simulink model "SWC_HALOUT_type"  (R2021b)
settings: Solver=FixedStepDiscrete  StartTime=0.0  StopTime=10.0  FixedStep=0.005  RelTol=1e-3
undefined symbols (not defined in the file): DIDLen_APPD, DIDLen_APPE, DIDLen_APPPedalZP, DIDLen_APSFunConfig, DIDLen_AutoLock, DIDLen_AutoWipHSpdEN, DIDLen_CALID, DIDLen_CDEODT, DIDLen_CLRDIST, DIDLen_DKCBLESta, DIDLen_DKCKey, DIDLen_DKCSta, DIDLen_DoorNFCAnchorSta, DIDLen_DRLDis, DIDLen_DynoMode, DIDLen_ECUNAME, DIDLen_FDDKCCoordXY, DIDLen_FMHTimer, DIDLen_LFLowPresThre, DIDLen_LFSensorID, DIDLen_LIDAAnchorSta, DIDLen_LRLowPresThre, DIDLen_LRSensorID, DIDLen_MILDIST, DIDLen_NUMPSATRIPSFLTMEMCLR, DIDLen_NVMPedalZP, DIDLen_OBDReq, DIDLen_ODOMETER, DIDLen_PKE, DIDLen_ProtocolId, DIDLen_PSA, DIDLen_QTYPSATRIPS, DIDLen_RFLowPresThre, DIDLen_RFSensorID, DIDLen_RRLowPresThre, DIDLen_RRSensorID, DIDLen_RUNTM, DIDLen_SensorMode, DIDLen_TestGroup, DIDLen_TireSize, DIDLen_TPMSLearnSta, DIDLen_TurnLampFLThreCurr, DIDLen_TurnLampFRThreCurr, DIDLen_TurnLampRLThreCurr, DIDLen_TurnLampRRThreCurr, DIDLen_UIDSta, DIDLen_USSConfig, DIDLen_UWBAnchorSta, DIDLen_VIN, DIDLen_VSS, DIDLen_WhlPres, DIDLen_WhlSensorBattSta, DIDLen_WhlTmp, DIDLen_WipRLSCmdCutFilter, DIDLen_WipRLSCmdHoldFilter, DIDLen_XWDMode, DIDNum_APPD, DIDNum_APPE, DIDNum_APPPedalZP, DIDNum_APSFunConfig ... (+504)
libraries: simulink x893, FVT_lib x320, hdlsllib x6, hcu_lib x5, halout x1
(part 2 of 11)

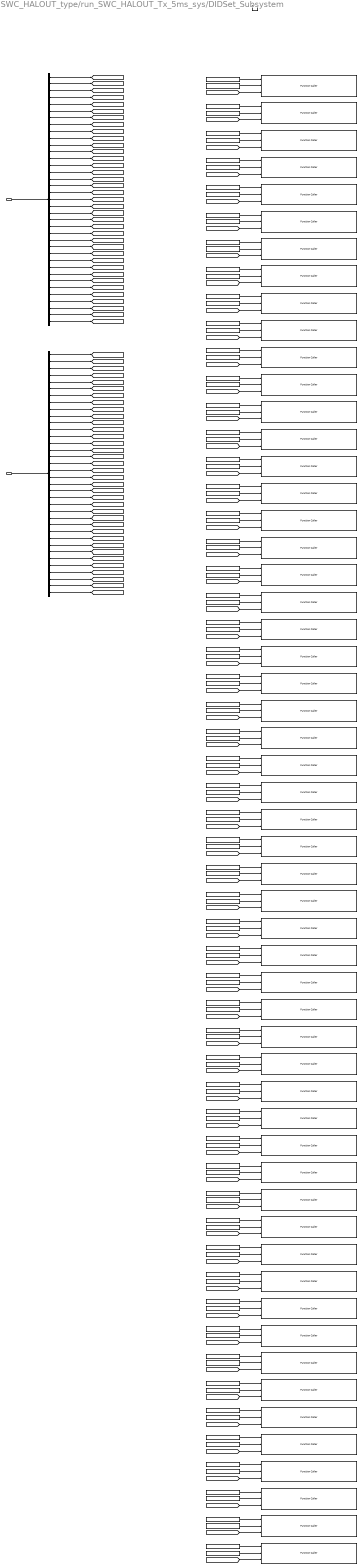
== system SWC_HALOUT_type/run_SWC_HALOUT_Tx_5ms_sys/DIDSet_Subsystem ==
  BOUTP_DIDSetData_outputs : Inport
  BHAL_DID_outputs : Inport  Port=2
  trig_SetDID : TriggerPort  TriggerType=function-call  VariantControl=(inherit)  PortDimensions=1
  DIDLen : Constant  Value=DIDNum_XWDMode
  DIDLen1 : Constant  Value=DIDNum_DKCKey
  DIDLen10 : Constant  Value=DIDNum_DRLDis
  DIDLen11 : Constant  Value=DIDNum_AutoWipHSpdEN
  DIDLen12 : Constant  Value=DIDNum_WipRLSCmdHoldFilter
  DIDLen13 : Constant  Value=DIDNum_WipRLSCmdCutFilter
  DIDLen14 : Constant  Value=DIDNum_LFSensorID
  DIDLen15 : Constant  Value=DIDNum_RFSensorID
  DIDLen16 : Constant  Value=DIDNum_LRSensorID
  DIDLen17 : Constant  Value=DIDNum_RRSensorID
  DIDLen18 : Constant  Value=DIDNum_WhlPres
  DIDLen19 : Constant  Value=DIDNum_WhlTmp
  DIDLen2 : Constant  Value=DIDNum_DynoMode
  DIDLen20 : Constant  Value=DIDNum_WhlSensorBattSta
  DIDLen21 : Constant  Value=DIDNum_LFLowPresThre
  DIDLen22 : Constant  Value=DIDNum_RFLowPresThre
  DIDLen23 : Constant  Value=DIDNum_LRLowPresThre
  DIDLen24 : Constant  Value=DIDNum_RRLowPresThre
  DIDLen25 : Constant  Value=DIDNum_SensorMode
  DIDLen26 : Constant  Value=DIDNum_TPMSLearnSta
  DIDLen27 : Constant  Value=DIDNum_USSConfig
  DIDLen28 : Constant  Value=DIDNum_TireSize
  DIDLen29 : Constant  Value=DIDNum_APSFunConfig
  DIDLen3 : Constant  Value=DIDNum_APPPedalZP
  DIDLen30 : Constant  Value=DIDNum_VSS
  DIDLen31 : Constant  Value=DIDNum_OBDReq
  DIDLen32 : Constant  Value=DIDNum_RUNTM
  DIDLen33 : Constant  Value=DIDNum_MILDIST
  DIDLen34 : Constant  Value=DIDNum_CLRDIST
  DIDLen35 : Constant  Value=DIDNum_APPD
  DIDLen36 : Constant  Value=DIDNum_APPE
  DIDLen37 : Constant  Value=DIDNum_ODOMETER
  DIDLen38 : Constant  Value=DIDNum_NUMPSATRIPSFLTMEMCLR
  DIDLen39 : Constant  Value=DIDNum_VIN
  DIDLen4 : Constant  Value=DIDNum_TurnLampFRThreCurr
  DIDLen40 : Constant  Value=DIDNum_CALID
  DIDLen41 : Constant  Value=DIDNum_ECUNAME
  DIDLen42 : Constant  Value=DIDNum_ProtocolId
  DIDLen43 : Constant  Value=DIDNum_TestGroup
  DIDLen44 : Constant  Value=DIDNum_PSA
  DIDLen45 : Constant  Value=DIDNum_PKE
  DIDLen46 : Constant  Value=DIDNum_CDEODT
  DIDLen47 : Constant  Value=DIDNum_QTYPSATRIPS
  DIDLen48 : Constant  Value=DIDNum_DKCSta
  DIDLen49 : Constant  Value=DIDNum_DKCBLESta
  DIDLen5 : Constant  Value=DIDNum_TurnLampRRThreCurr
  DIDLen50 : Constant  Value=DIDNum_UWBAnchorSta
  DIDLen51 : Constant  Value=DIDNum_LIDAAnchorSta
  DIDLen52 : Constant  Value=DIDNum_DoorNFCAnchorSta
  DIDLen53 : Constant  Value=DIDNum_UIDSta
  DIDLen54 : Constant  Value=DIDNum_FDDKCCoordXY
  DIDLen6 : Constant  Value=DIDNum_TurnLampFLThreCurr
  DIDLen7 : Constant  Value=DIDNum_TurnLampRLThreCurr
  DIDLen8 : Constant  Value=DIDNum_FMHTimer
  DIDLen9 : Constant  Value=DIDNum_AutoLock
  DIDNum : Constant  Value=DIDLen_XWDMode
  DIDNum1 : Constant  Value=DIDLen_DKCKey
  DIDNum10 : Constant  Value=DIDLen_DRLDis
  DIDNum11 : Constant  Value=DIDLen_AutoWipHSpdEN
  DIDNum12 : Constant  Value=DIDLen_WipRLSCmdHoldFilter
  DIDNum13 : Constant  Value=DIDLen_WipRLSCmdCutFilter
  DIDNum14 : Constant  Value=DIDLen_LFSensorID
  DIDNum15 : Constant  Value=DIDLen_RFSensorID
  DIDNum16 : Constant  Value=DIDLen_LRSensorID
  DIDNum17 : Constant  Value=DIDLen_RRSensorID
  DIDNum18 : Constant  Value=DIDLen_WhlPres
  DIDNum19 : Constant  Value=DIDLen_WhlTmp
  DIDNum2 : Constant  Value=DIDLen_DynoMode
  DIDNum20 : Constant  Value=DIDLen_WhlSensorBattSta
  DIDNum21 : Constant  Value=DIDLen_LFLowPresThre
  DIDNum22 : Constant  Value=DIDLen_RFLowPresThre
  DIDNum23 : Constant  Value=DIDLen_LRLowPresThre
  DIDNum24 : Constant  Value=DIDLen_RRLowPresThre
  DIDNum25 : Constant  Value=DIDLen_SensorMode
  DIDNum26 : Constant  Value=DIDLen_TPMSLearnSta
  DIDNum27 : Constant  Value=DIDLen_USSConfig
  DIDNum28 : Constant  Value=DIDLen_TireSize
  DIDNum29 : Constant  Value=DIDLen_APSFunConfig
  DIDNum3 : Constant  Value=DIDLen_APPPedalZP
  DIDNum30 : Constant  Value=DIDLen_VSS
  DIDNum31 : Constant  Value=DIDLen_OBDReq
  DIDNum32 : Constant  Value=DIDLen_RUNTM
  DIDNum33 : Constant  Value=DIDLen_MILDIST
  DIDNum34 : Constant  Value=DIDLen_CLRDIST
  DIDNum35 : Constant  Value=DIDLen_APPD
  DIDNum36 : Constant  Value=DIDLen_APPE
  DIDNum37 : Constant  Value=DIDLen_ODOMETER
  DIDNum38 : Constant  Value=DIDLen_NUMPSATRIPSFLTMEMCLR
  DIDNum39 : Constant  Value=DIDLen_VIN
  DIDNum4 : Constant  Value=DIDLen_TurnLampFRThreCurr
  DIDNum40 : Constant  Value=DIDLen_CALID
  DIDNum41 : Constant  Value=DIDLen_ECUNAME
  DIDNum42 : Constant  Value=DIDLen_ProtocolId
  DIDNum43 : Constant  Value=DIDLen_TestGroup
  DIDNum44 : Constant  Value=DIDLen_PSA
  DIDNum45 : Constant  Value=DIDLen_PKE
  DIDNum46 : Constant  Value=DIDLen_CDEODT
  DIDNum47 : Constant  Value=DIDLen_QTYPSATRIPS
  DIDNum48 : Constant  Value=DIDLen_DKCSta
  DIDNum49 : Constant  Value=DIDLen_DKCBLESta
  DIDNum5 : Constant  Value=DIDLen_TurnLampRRThreCurr
  DIDNum50 : Constant  Value=DIDLen_UWBAnchorSta
  DIDNum51 : Constant  Value=DIDLen_LIDAAnchorSta
  DIDNum52 : Constant  Value=DIDLen_DoorNFCAnchorSta
  DIDNum53 : Constant  Value=DIDLen_UIDSta
  DIDNum54 : Constant  Value=DIDLen_FDDKCCoordXY
  DIDNum6 : Constant  Value=DIDLen_TurnLampFLThreCurr
  DIDNum7 : Constant  Value=DIDLen_TurnLampRLThreCurr
  DIDNum8 : Constant  Value=DIDLen_FMHTimer
  DIDNum9 : Constant  Value=DIDLen_AutoLock
  R_DIDWriteCDD_CSOP_DIDSet_APPD : FunctionCaller  FunctionPrototype=R_DIDWriteCDD_CSOP_DIDSet_APPD(u16_DIDNum_APPD,u16_DIDLen_APPD,u8_APPD)  InputArgumentSpecifications=uint16(1), uint16(1), uint8(1)
  R_DIDWriteCDD_CSOP_DIDSet_APPE : FunctionCaller  FunctionPrototype=R_DIDWriteCDD_CSOP_DIDSet_APPE(u16_DIDNum_APPE,u16_DIDLen_APPE,u8_APPE)  InputArgumentSpecifications=uint16(1), uint16(1), uint8(1)
  R_DIDWriteCDD_CSOP_DIDSet_APPPedalZP : FunctionCaller  FunctionPrototype=R_DIDWriteCDD_CSOP_DIDSet_APPPedalZP(u16_DIDNum_APPPedalZP,u16_DIDLen_APPPedalZP,u8Array3_APPPedalZP)  InputArgumentSpecifications=uint16(1), uint16(1), uint8([1;1;1])
  R_DIDWriteCDD_CSOP_DIDSet_APSFunConfig : FunctionCaller  FunctionPrototype=R_DIDWriteCDD_CSOP_DIDSet_APSFunConfig(u16_DIDNum_APSFunConfig,u16_DIDLen_APSFunConfig,u8Array16_APSFunConfig)  InputArgumentSpecifications=uint16(1), uint16(1), uint8([1;1;1;1;1;1;1;1;1;1;1;1;1;1;1;1])
  R_DIDWriteCDD_CSOP_DIDSet_AutoLock : FunctionCaller  FunctionPrototype=R_DIDWriteCDD_CSOP_DIDSet_AutoLock(u16_DIDNum_AutoLock,u16_DIDLen_AutoLock,u8_AutoLock)  InputArgumentSpecifications=uint16(1), uint16(1), uint8(1)
  R_DIDWriteCDD_CSOP_DIDSet_AutoWipHSpdEN : FunctionCaller  FunctionPrototype=R_DIDWriteCDD_CSOP_DIDSet_AutoWipHSpdEN(u16_DIDNum_AutoWipHSpdEN,u16_DIDLen_AutoWipHSpdEN,u8_AutoWipHSpdEN)  InputArgumentSpecifications=uint16(1), uint16(1), uint8(1)
  R_DIDWriteCDD_CSOP_DIDSet_CALID : FunctionCaller  FunctionPrototype=R_DIDWriteCDD_CSOP_DIDSet_CALID(u16_DIDNum_CALID,u16_DIDLen_CALID,u8Array16_CALID)  InputArgumentSpecifications=uint16(1), uint16(1), uint8([1;1;1;1;1;1;1;1;1;1;1;1;1;1;1;1])
  R_DIDWriteCDD_CSOP_DIDSet_CDEODT : FunctionCaller  FunctionPrototype=R_DIDWriteCDD_CSOP_DIDSet_CDEODT(u16_DIDNum_CDEODT,u16_DIDLen_CDEODT,u8Array8_CDEODT)  InputArgumentSpecifications=uint16(1), uint16(1), uint8([1;1;1;1;1;1;1;1])
  R_DIDWriteCDD_CSOP_DIDSet_CLRDIST : FunctionCaller  FunctionPrototype=R_DIDWriteCDD_CSOP_DIDSet_CLRDIST(u16_DIDNum_CLRDIST,u16_DIDLen_CLRDIST,u8Array2_CLRDIST)  InputArgumentSpecifications=uint16(1), uint16(1), uint8([1;1])
  R_DIDWriteCDD_CSOP_DIDSet_DKCBLESta : FunctionCaller  FunctionPrototype=R_DIDWriteCDD_CSOP_DIDSet_DKCBLESta(u16_DIDNum_DKCBLESta,u16_DIDLen_DKCBLESta,u8Array2_DKCBLESta)  InputArgumentSpecifications=uint16(1), uint16(1), uint8([1;1])
  R_DIDWriteCDD_CSOP_DIDSet_DKCKey : FunctionCaller  FunctionPrototype=R_DIDWriteCDD_CSOP_DIDSet_DKCKey(u16_DIDNum_DKCKey,u16_DIDLen_DKCKey,u8Array8_DKCKey)  InputArgumentSpecifications=uint16(1), uint16(1), uint8([1;1;1;1;1;1;1;1])
  R_DIDWriteCDD_CSOP_DIDSet_DKCSta : FunctionCaller  FunctionPrototype=R_DIDWriteCDD_CSOP_DIDSet_DKCSta(u16_DIDNum_DKCSta,u16_DIDLen_DKCSta,u8Array2_DKCSta)  InputArgumentSpecifications=uint16(1), uint16(1), uint8([1;1])
  R_DIDWriteCDD_CSOP_DIDSet_DRLDis : FunctionCaller  FunctionPrototype=R_DIDWriteCDD_CSOP_DIDSet_DRLDis(u16_DIDNum_DRLDis,u16_DIDLen_DRLDis,u8_DRLDis)  InputArgumentSpecifications=uint16(1), uint16(1), uint8(1)
  R_DIDWriteCDD_CSOP_DIDSet_DoorNFCAnchorSta : FunctionCaller  FunctionPrototype=R_DIDWriteCDD_CSOP_DIDSet_DoorNFCAnchorSta(u16_DIDNum_DoorNFCAnchorSta,u16_DIDLen_DoorNFCAnchorSta,u8Array21_DoorNFCAnchorSta)  InputArgumentSpecifications=uint16(1), uint16(1), uint8([1;1;1;1;1;1;1;1;1;1;1;1;1;1;1;1;1;1;1;1;1])
  R_DIDWriteCDD_CSOP_DIDSet_DynoMode : FunctionCaller  FunctionPrototype=R_DIDWriteCDD_CSOP_DIDSet_DynoMode(u16_DIDNum_DynoMode,u16_DIDLen_DynoMode,u8_DynoMode)  InputArgumentSpecifications=uint16(1), uint16(1), uint8(1)
  R_DIDWriteCDD_CSOP_DIDSet_ECUNAME : FunctionCaller  FunctionPrototype=R_DIDWriteCDD_CSOP_DIDSet_ECUNAME(u16_DIDNum_ECUNAME,u16_DIDLen_ECUNAME,u8Array20_ECUNAME)  InputArgumentSpecifications=uint16(1), uint16(1), uint8([1;1;1;1;1;1;1;1;1;1;1;1;1;1;1;1;1;1;1;1])
  R_DIDWriteCDD_CSOP_DIDSet_FDDKCCoordXY : FunctionCaller  FunctionPrototype=R_DIDWriteCDD_CSOP_DIDSet_FDDKCCoordXY(u16_DIDNum_FDDKCCoordXY,u16_DIDLen_FDDKCCoordXY,u8Array3_FDDKCCoordXY)  InputArgumentSpecifications=uint16(1), uint16(1), uint8([1;1;1])
  R_DIDWriteCDD_CSOP_DIDSet_FMHTimer : FunctionCaller  FunctionPrototype=R_DIDWriteCDD_CSOP_DIDSet_FMHTimer(u16_DIDNum_FMHTimer,u16_DIDLen_FMHTimer,u8_FMHTimer)  InputArgumentSpecifications=uint16(1), uint16(1), uint8(1)
  R_DIDWriteCDD_CSOP_DIDSet_LFLowPresThre : FunctionCaller  FunctionPrototype=R_DIDWriteCDD_CSOP_DIDSet_LFLowPresThre(u16_DIDNum_LFLowPresThre,u16_DIDLen_LFLowPresThre,u8_LFLowPresThre)  InputArgumentSpecifications=uint16(1), uint16(1), uint8(1)
  R_DIDWriteCDD_CSOP_DIDSet_LFSensorID : FunctionCaller  FunctionPrototype=R_DIDWriteCDD_CSOP_DIDSet_LFSensorID(u16_DIDNum_LFSensorID,u16_DIDLen_LFSensorID,u8Array4_LFSensorID)  InputArgumentSpecifications=uint16(1), uint16(1), uint8([1;1;1;1])
  R_DIDWriteCDD_CSOP_DIDSet_LIDAAnchorSta : FunctionCaller  FunctionPrototype=R_DIDWriteCDD_CSOP_DIDSet_LIDAAnchorSta(u16_DIDNum_LIDAAnchorSta,u16_DIDLen_LIDAAnchorSta,u8Array21_LIDAAnchorSta)  InputArgumentSpecifications=uint16(1), uint16(1), uint8([1;1;1;1;1;1;1;1;1;1;1;1;1;1;1;1;1;1;1;1;1])
  R_DIDWriteCDD_CSOP_DIDSet_LRLowPresThre : FunctionCaller  FunctionPrototype=R_DIDWriteCDD_CSOP_DIDSet_LRLowPresThre(u16_DIDNum_LRLowPresThre,u16_DIDLen_LRLowPresThre,u8_LRLowPresThre)  InputArgumentSpecifications=uint16(1), uint16(1), uint8(1)
  R_DIDWriteCDD_CSOP_DIDSet_LRSensorID : FunctionCaller  FunctionPrototype=R_DIDWriteCDD_CSOP_DIDSet_LRSensorID(u16_DIDNum_LRSensorID,u16_DIDLen_LRSensorID,u8Array4_LRSensorID)  InputArgumentSpecifications=uint16(1), uint16(1), uint8([1;1;1;1])
  R_DIDWriteCDD_CSOP_DIDSet_MILDIST : FunctionCaller  FunctionPrototype=R_DIDWriteCDD_CSOP_DIDSet_MILDIST(u16_DIDNum_MILDIST,u16_DIDLen_MILDIST,u8Array2_MILDIST)  InputArgumentSpecifications=uint16(1), uint16(1), uint8([1;1])
  R_DIDWriteCDD_CSOP_DIDSet_NUMPSATRIPSFLTMEMCLR : FunctionCaller  FunctionPrototype=R_DIDWriteCDD_CSOP_DIDSet_NUMPSATRIPSFLTMEMCLR(u16_DIDNum_NUMPSATRIPSFLTMEMCLR,u16_DIDLen_NUMPSATRIPSFLTMEMCLR,u8Array2_NUMPSATRIPSFLTMEMCLR)  InputArgumentSpecifications=uint16(1), uint16(1), uint8([1;1])
  R_DIDWriteCDD_CSOP_DIDSet_OBDReq : FunctionCaller  FunctionPrototype=R_DIDWriteCDD_CSOP_DIDSet_OBDReq(u16_DIDNum_OBDReq,u16_DIDLen_OBDReq,u8_OBDReq)  InputArgumentSpecifications=uint16(1), uint16(1), uint8(1)
  R_DIDWriteCDD_CSOP_DIDSet_ODOMETER : FunctionCaller  FunctionPrototype=R_DIDWriteCDD_CSOP_DIDSet_ODOMETER(u16_DIDNum_ODOMETER,u16_DIDLen_ODOMETER,u8Array4_ODOMETER)  InputArgumentSpecifications=uint16(1), uint16(1), uint8([1;1;1;1])
  R_DIDWriteCDD_CSOP_DIDSet_PKE : FunctionCaller  FunctionPrototype=R_DIDWriteCDD_CSOP_DIDSet_PKE(u16_DIDNum_PKE,u16_DIDLen_PKE,u8Array8_PKE)  InputArgumentSpecifications=uint16(1), uint16(1), uint8([1;1;1;1;1;1;1;1])
  R_DIDWriteCDD_CSOP_DIDSet_PSA : FunctionCaller  FunctionPrototype=R_DIDWriteCDD_CSOP_DIDSet_PSA(u16_DIDNum_PSA,u16_DIDLen_PSA,u8Array24_PSA)  InputArgumentSpecifications=uint16(1), uint16(1), uint8([1;1;1;1;1;1;1;1;1;1;1;1;1;1;1;1;1;1;1;1;1;1;1;1])
  R_DIDWriteCDD_CSOP_DIDSet_ProtocolId : FunctionCaller  FunctionPrototype=R_DIDWriteCDD_CSOP_DIDSet_ProtocolId(u16_DIDNum_ProtocolId,u16_DIDLen_ProtocolId,u8_ProtocolId)  InputArgumentSpecifications=uint16(1), uint16(1), uint8(1)
  R_DIDWriteCDD_CSOP_DIDSet_QTYPSATRIPS : FunctionCaller  FunctionPrototype=R_DIDWriteCDD_CSOP_DIDSet_QTYPSATRIPS(u16_DIDNum_QTYPSATRIPS,u16_DIDLen_QTYPSATRIPS,u8Array8_QTYPSATRIPS)  InputArgumentSpecifications=uint16(1), uint16(1), uint8([1;1;1;1;1;1;1;1])
  R_DIDWriteCDD_CSOP_DIDSet_RFLowPresThre : FunctionCaller  FunctionPrototype=R_DIDWriteCDD_CSOP_DIDSet_RFLowPresThre(u16_DIDNum_RFLowPresThre,u16_DIDLen_RFLowPresThre,u8_RFLowPresThre)  InputArgumentSpecifications=uint16(1), uint16(1), uint8(1)
  R_DIDWriteCDD_CSOP_DIDSet_RFSensorID : FunctionCaller  FunctionPrototype=R_DIDWriteCDD_CSOP_DIDSet_RFSensorID(u16_DIDNum_RFSensorID,u16_DIDLen_RFSensorID,u8Array4_RFSensorID)  InputArgumentSpecifications=uint16(1), uint16(1), uint8([1;1;1;1])
  R_DIDWriteCDD_CSOP_DIDSet_RRLowPresThre : FunctionCaller  FunctionPrototype=R_DIDWriteCDD_CSOP_DIDSet_RRLowPresThre(u16_DIDNum_RRLowPresThre,u16_DIDLen_RRLowPresThre,u8_RRLowPresThre)  InputArgumentSpecifications=uint16(1), uint16(1), uint8(1)
  R_DIDWriteCDD_CSOP_DIDSet_RRSensorID : FunctionCaller  FunctionPrototype=R_DIDWriteCDD_CSOP_DIDSet_RRSensorID(u16_DIDNum_RRSensorID,u16_DIDLen_RRSensorID,u8Array4_RRSensorID)  InputArgumentSpecifications=uint16(1), uint16(1), uint8([1;1;1;1])
  R_DIDWriteCDD_CSOP_DIDSet_RUNTM : FunctionCaller  FunctionPrototype=R_DIDWriteCDD_CSOP_DIDSet_RUNTM(u16_DIDNum_RUNTM,u16_DIDLen_RUNTM,u8Array2_RUNTM)  InputArgumentSpecifications=uint16(1), uint16(1), uint8([1;1])
  R_DIDWriteCDD_CSOP_DIDSet_SensorMode : FunctionCaller  FunctionPrototype=R_DIDWriteCDD_CSOP_DIDSet_SensorMode(u16_DIDNum_SensorMode,u16_DIDLen_SensorMode,u8_SensorMode)  InputArgumentSpecifications=uint16(1), uint16(1), uint8(1)
  R_DIDWriteCDD_CSOP_DIDSet_TPMSLearnSta : FunctionCaller  FunctionPrototype=R_DIDWriteCDD_CSOP_DIDSet_TPMSLearnSta(u16_DIDNum_TPMSLearnSta,u16_DIDLen_TPMSLearnSta,u8_TPMSLearnSta)  InputArgumentSpecifications=uint16(1), uint16(1), uint8(1)
  R_DIDWriteCDD_CSOP_DIDSet_TestGroup : FunctionCaller  FunctionPrototype=R_DIDWriteCDD_CSOP_DIDSet_TestGroup(u16_DIDNum_TestGroup,u16_DIDLen_TestGroup,u8Array12_TestGroup)  InputArgumentSpecifications=uint16(1), uint16(1), uint8([1;1;1;1;1;1;1;1;1;1;1;1])
  R_DIDWriteCDD_CSOP_DIDSet_TireSize : FunctionCaller  FunctionPrototype=R_DIDWriteCDD_CSOP_DIDSet_TireSize(u16_DIDNum_TireSize,u16_DIDLen_TireSize,u8Array16_TireSize)  InputArgumentSpecifications=uint16(1), uint16(1), uint8([1;1;1;1;1;1;1;1;1;1;1;1;1;1;1;1])
  R_DIDWriteCDD_CSOP_DIDSet_TurnLampFLThreCurr : FunctionCaller  FunctionPrototype=R_DIDWriteCDD_CSOP_DIDSet_TurnLampFLThreCurr(u16_DIDNum_TurnLampFLThreCurr,u16_DIDLen_TurnLampFLThreCurr,u8_TurnLampFLThreCurr)  InputArgumentSpecifications=uint16(1), uint16(1), uint8(1)
  R_DIDWriteCDD_CSOP_DIDSet_TurnLampFRThreCurr : FunctionCaller  FunctionPrototype=R_DIDWriteCDD_CSOP_DIDSet_TurnLampFRThreCurr(u16_DIDNum_TurnLampFRThreCurr,u16_DIDLen_TurnLampFRThreCurr,u8_TurnLampFRThreCurr)  InputArgumentSpecifications=uint16(1), uint16(1), uint8(1)
  R_DIDWriteCDD_CSOP_DIDSet_TurnLampRLThreCurr : FunctionCaller  FunctionPrototype=R_DIDWriteCDD_CSOP_DIDSet_TurnLampRLThreCurr(u16_DIDNum_TurnLampRLThreCurr,u16_DIDLen_TurnLampRLThreCurr,u8_TurnLampRLThreCurr)  InputArgumentSpecifications=uint16(1), uint16(1), uint8(1)
  R_DIDWriteCDD_CSOP_DIDSet_TurnLampRRThreCurr : FunctionCaller  FunctionPrototype=R_DIDWriteCDD_CSOP_DIDSet_TurnLampRRThreCurr(u16_DIDNum_TurnLampRRThreCurr,u16_DIDLen_TurnLampRRThreCurr,u8_TurnLampRRThreCurr)  InputArgumentSpecifications=uint16(1), uint16(1), uint8(1)
  R_DIDWriteCDD_CSOP_DIDSet_UIDSta : FunctionCaller  FunctionPrototype=R_DIDWriteCDD_CSOP_DIDSet_UIDSta(u16_DIDNum_UIDSta,u16_DIDLen_UIDSta,u8Array26_UIDSta)  InputArgumentSpecifications=uint16(1), uint16(1), uint8([1;1;1;1;1;1;1;1;1;1;1;1;1;1;1;1;1;1;1;1;1;1;1;1;1;1])
  R_DIDWriteCDD_CSOP_DIDSet_USSConfig : FunctionCaller  FunctionPrototype=R_DIDWriteCDD_CSOP_DIDSet_USSConfig(u16_DIDNum_USSConfig,u16_DIDLen_USSConfig,u8Array16_USSConfig)  InputArgumentSpecifications=uint16(1), uint16(1), uint8([1;1;1;1;1;1;1;1;1;1;1;1;1;1;1;1])
  R_DIDWriteCDD_CSOP_DIDSet_UWBAnchorSta : FunctionCaller  FunctionPrototype=R_DIDWriteCDD_CSOP_DIDSet_UWBAnchorSta(u16_DIDNum_UWBAnchorSta,u16_DIDLen_UWBAnchorSta,u8Array93_UWBAnchorSta)  InputArgumentSpecifications=uint16(1), uint16(1), uint8([1;1;1;1;1;1;1;1;1;1;1;1;1;1;1;1;1;1;1;1;1;1;1;1;1;1;1;1;1;1;1;1;1;1;1;1;1;1;1;1;1;1;1;1;1;1;1;1;1;1;1;1;1;1;1;1;1;1;1;1;1;1;1;1;1;1;1;1;1;1;1;1;1;1;1;1;1;1;1;1;1;1;1;1;1;1;1;1;1;1;1;1;1])
  R_DIDWriteCDD_CSOP_DIDSet_VIN : FunctionCaller  FunctionPrototype=R_DIDWriteCDD_CSOP_DIDSet_VIN(u16_DIDNum_VIN,u16_DIDLen_VIN,u8Array17_VIN)  InputArgumentSpecifications=uint16(1), uint16(1), uint8([1;1;1;1;1;1;1;1;1;1;1;1;1;1;1;1;1])
  R_DIDWriteCDD_CSOP_DIDSet_VSS : FunctionCaller  FunctionPrototype=R_DIDWriteCDD_CSOP_DIDSet_VSS(u16_DIDNum_VSS,u16_DIDLen_VSS,u8_VSS)  InputArgumentSpecifications=uint16(1), uint16(1), uint8(1)
  R_DIDWriteCDD_CSOP_DIDSet_WhlPres : FunctionCaller  FunctionPrototype=R_DIDWriteCDD_CSOP_DIDSet_WhlPres(u16_DIDNum_WhlPres,u16_DIDLen_WhlPres,u8Array4_WhlPres)  InputArgumentSpecifications=uint16(1), uint16(1), uint8([1;1;1;1])
  R_DIDWriteCDD_CSOP_DIDSet_WhlSensorBattSta : FunctionCaller  FunctionPrototype=R_DIDWriteCDD_CSOP_DIDSet_WhlSensorBattSta(u16_DIDNum_WhlSensorBattSta,u16_DIDLen_WhlSensorBattSta,u8_WhlSensorBattSta)  InputArgumentSpecifications=uint16(1), uint16(1), uint8(1)
  R_DIDWriteCDD_CSOP_DIDSet_WhlTmp : FunctionCaller  FunctionPrototype=R_DIDWriteCDD_CSOP_DIDSet_WhlTmp(u16_DIDNum_WhlTmp,u16_DIDLen_WhlTmp,u8Array4_WhlTmp)  InputArgumentSpecifications=uint16(1), uint16(1), uint8([1;1;1;1])
  R_DIDWriteCDD_CSOP_DIDSet_WipRLSCmdCutFilter : FunctionCaller  FunctionPrototype=R_DIDWriteCDD_CSOP_DIDSet_WipRLSCmdCutFilter(u16_DIDNum_WipRLSCmdCutFilter,u16_DIDLen_WipRLSCmdCutFilter,u8_WipRLSCmdCutFilter)  InputArgumentSpecifications=uint16(1), uint16(1), uint8(1)
  R_DIDWriteCDD_CSOP_DIDSet_WipRLSCmdHoldFilter : FunctionCaller  FunctionPrototype=R_DIDWriteCDD_CSOP_DIDSet_WipRLSCmdHoldFilter(u16_DIDNum_WipRLSCmdHoldFilter,u16_DIDLen_WipRLSCmdHoldFilter,u8_WipRLSCmdHoldFilter)  InputArgumentSpecifications=uint16(1), uint16(1), uint8(1)
  R_DIDWriteCDD_CSOP_DIDSet_XWDMode : FunctionCaller  FunctionPrototype=R_DIDWriteCDD_CSOP_DIDSet_XWDMode(u16_DIDNum_XWDMode,u16_DIDLen_XWDMode,u8_XWDMode)  InputArgumentSpecifications=uint16(1), uint16(1), uint8(1)
  bus_selector : BusSelector  OutputSignals=VHAL_DIDSetAPPPedalZP_raw8,VHAL_DIDSetLFSensorID_raw8,VHAL_DIDSetRFSensorID_raw8,VHAL_DIDSetLRSensorID_raw8,VHAL_DIDSetRRSensorID_raw8,VHAL_DIDSetWhlPres_raw8,VHAL_DIDSetWhlTmp_raw8,VHAL_DIDSetWhlSensorBattSta_raw8,VHAL_DIDSetLFLowPresThre_raw8,VHAL_DIDSetRFLowPresThre_raw8,VHAL_DIDSetLRLowPresThre_raw8,VHAL_DIDSetRRLowPresThre_raw8,VHAL_DIDSetSensorMode_raw8,VHAL_DIDSetTPMSLearnSta_raw8,VHAL_DIDSetVSS_raw8,VHAL_DIDSetRUNTM_raw8,VHAL_DIDSetMILDIST_raw8,VHAL_DIDSetCLRDIST_raw8,VHAL_DIDSetAPPD_raw8,VHAL_DIDSetAPPE_raw8,VHAL_DIDSetODOMETER_raw8,VHAL_DIDSetNUMPSATRIPSFLTMEMCLR_raw8,VHAL_DIDSetVIN_raw8,VHAL_DIDSetCALID_raw8,VHAL_DIDSetECUNAME_raw8,VHAL_DIDSetProtocolId_raw8,VHAL_DIDSetPSA_raw8,VHAL_DIDSetPKE_raw8,VHAL_DIDSetCDEODT_raw8,VHAL_DIDSetQTYPSATRIPS_raw8,VHAL_DIDSetDKCSta_raw8,VHAL_DIDSetDKCBLESta_raw8,VHAL_DIDSetUWBAnchorSta_raw8,VHAL_DIDSetLIDAAnchorSta_raw8,VHAL_DIDSetDoorNFCAnchorSta_raw8,VHAL_DIDSetUIDSta_raw8,VHAL_DIDSetFDDKCCoordXY_raw8
  bus_selector1 : BusSelector  OutputSignals=VHAL_DIDStaXWDMode_raw,VHAL_XWDMode_raw,VHAL_DIDStaDKCKey_raw,VHAL_DKCKey_raw,VHAL_DIDStaDynoMode_raw,VHAL_DynoMode_raw,VHAL_DIDStaTurnLampFRThreCurr_raw,VHAL_TurnLampFRThreCurr_raw,VHAL_DIDStaTurnLampRRThreCurr_raw,VHAL_TurnLampRRThreCurr_raw,VHAL_DIDStaTurnLampFLThreCurr_raw,VHAL_TurnLampFLThreCurr_raw,VHAL_DIDStaTurnLampRLThreCurr_raw,VHAL_TurnLampRLThreCurr_raw,VHAL_DIDStaFMHTimer_raw,VHAL_FMHTimer_raw,VHAL_DIDStaAutoLock_raw,VHAL_AutoLock_raw,VHAL_DIDStaDRLDis_raw,VHAL_DRLDis_raw,VHAL_DIDStaAutoWipHSpdEN_raw,VHAL_AutoWipHSpdEN_raw,VHAL_DIDStaWipRLSCmdHoldFilter_raw,VHAL_WipRLSCmdHoldFilter_raw,VHAL_DIDStaWipRLSCmdCutFilter_raw,VHAL_WipRLSCmdCutFilter_raw,VHAL_DIDStaUSSConfig_raw,VHAL_USSConfig_raw,VHAL_DIDStaTireSize_raw,VHAL_TireSize_raw,VHAL_DIDStaAPSFunConfig_raw,VHAL_APSFunConfig_raw,VHAL_DIDStaOBDReq_raw,VHAL_OBDReq_raw,VHAL_DIDStaTestGroup_raw,VHAL_TestGroup_raw
  wires:
  bus_selector/1 -> [u8Array3_APPPedalZP]  "<VHAL_DIDSetAPPPedalZP_raw8>"
  bus_selector/2 -> [u8Array4_LFSensorID]  "<VHAL_DIDSetLFSensorID_raw8>"
  bus_selector/3 -> [u8Array4_RFSensorID]  "<VHAL_DIDSetRFSensorID_raw8>"
  bus_selector/4 -> [u8Array4_LRSensorID]  "<VHAL_DIDSetLRSensorID_raw8>"
  bus_selector/5 -> [u8Array4_RRSensorID]  "<VHAL_DIDSetRRSensorID_raw8>"
  bus_selector/6 -> [u8Array4_WhlPres]  "<VHAL_DIDSetWhlPres_raw8>"
  bus_selector/7 -> [u8Array4_WhlTmp]  "<VHAL_DIDSetWhlTmp_raw8>"
  bus_selector/8 -> [u8_WhlSensorBattSta]  "<VHAL_DIDSetWhlSensorBattSta_raw8>"
  bus_selector/9 -> [u8_LFLowPresThre]  "<VHAL_DIDSetLFLowPresThre_raw8>"
  bus_selector/10 -> [u8_RFLowPresThre]  "<VHAL_DIDSetRFLowPresThre_raw8>"
  bus_selector/11 -> [u8_LRLowPresThre]  "<VHAL_DIDSetLRLowPresThre_raw8>"
  bus_selector/12 -> [u8_RRLowPresThre]  "<VHAL_DIDSetRRLowPresThre_raw8>"
  bus_selector/13 -> [u8_SensorMode]  "<VHAL_DIDSetSensorMode_raw8>"
  bus_selector/14 -> [u8_TPMSLearnSta]  "<VHAL_DIDSetTPMSLearnSta_raw8>"
  bus_selector/15 -> [u8_VSS]  "<VHAL_DIDSetVSS_raw8>"
  bus_selector/16 -> [u8Array2_RUNTM]  "<VHAL_DIDSetRUNTM_raw8>"
  bus_selector/17 -> [u8Array2_MILDIST]  "<VHAL_DIDSetMILDIST_raw8>"
  bus_selector/18 -> [u8Array2_CLRDIST]  "<VHAL_DIDSetCLRDIST_raw8>"
  bus_selector/19 -> [u8_APPD]  "<VHAL_DIDSetAPPD_raw8>"
  bus_selector/20 -> [u8_APPE]  "<VHAL_DIDSetAPPE_raw8>"
  bus_selector/21 -> [u8Array4_ODOMETER]  "<VHAL_DIDSetODOMETER_raw8>"
  bus_selector/22 -> [u8Array2_NUMPSATRIPSFLTMEMCLR]  "<VHAL_DIDSetNUMPSATRIPSFLTMEMCLR_raw8>"
  bus_selector/23 -> [u8Array17_VIN]  "<VHAL_DIDSetVIN_raw8>"
  bus_selector/24 -> [u8Array16_CALID]  "<VHAL_DIDSetCALID_raw8>"
  bus_selector/25 -> [u8Array20_ECUNAME]  "<VHAL_DIDSetECUNAME_raw8>"
  bus_selector/26 -> [u8_ProtocolId]  "<VHAL_DIDSetProtocolId_raw8>"
  bus_selector/27 -> [u8Array24_PSA]  "<VHAL_DIDSetPSA_raw8>"
  bus_selector/28 -> [u8Array8_PKE]  "<VHAL_DIDSetPKE_raw8>"
  bus_selector/29 -> [u8Array8_CDEODT]  "<VHAL_DIDSetCDEODT_raw8>"
  bus_selector/30 -> [u8Array8_QTYPSATRIPS]  "<VHAL_DIDSetQTYPSATRIPS_raw8>"
  bus_selector/31 -> [u8Array2_DKCSta]  "<VHAL_DIDSetDKCSta_raw8>"
  bus_selector/32 -> [u8Array2_DKCBLESta]  "<VHAL_DIDSetDKCBLESta_raw8>"
  bus_selector/33 -> [u8Array93_UWBAnchorSta]  "<VHAL_DIDSetUWBAnchorSta_raw8>"
  bus_selector/34 -> [u8Array21_LIDAAnchorSta]  "<VHAL_DIDSetLIDAAnchorSta_raw8>"
  bus_selector/35 -> [u8Array21_DoorNFCAnchorSta]  "<VHAL_DIDSetDoorNFCAnchorSta_raw8>"
  bus_selector/36 -> [u8Array26_UIDSta]  "<VHAL_DIDSetUIDSta_raw8>"
  bus_selector/37 -> [u8Array3_FDDKCCoordXY]  "<VHAL_DIDSetFDDKCCoordXY_raw8>"
  BOUTP_DIDSetData_outputs/1 -> bus_selector/1
  bus_selector1/1 -> [u8_DIDSta_XWDMode]  "<VHAL_DIDStaXWDMode_raw>"
  bus_selector1/2 -> [u8_XWDMode]  "<VHAL_XWDMode_raw>"
  bus_selector1/3 -> [u8_DIDSta_DKCKey]  "<VHAL_DIDStaDKCKey_raw>"
  bus_selector1/4 -> [u8Array8_DKCKey]  "<VHAL_DKCKey_raw>"
  bus_selector1/5 -> [u8_DIDSta_DynoMode]  "<VHAL_DIDStaDynoMode_raw>"
  bus_selector1/6 -> [u8_DynoMode]  "<VHAL_DynoMode_raw>"
  bus_selector1/7 -> [u8_DIDSta_TurnLampFRThreCurr]  "<VHAL_DIDStaTurnLampFRThreCurr_raw>"
  bus_selector1/8 -> [u8_TurnLampFRThreCurr]  "<VHAL_TurnLampFRThreCurr_raw>"
  bus_selector1/9 -> [u8_DIDSta_TurnLampRRThreCurr]  "<VHAL_DIDStaTurnLampRRThreCurr_raw>"
  bus_selector1/10 -> [u8_TurnLampRRThreCurr]  "<VHAL_TurnLampRRThreCurr_raw>"
  bus_selector1/11 -> [u8_DIDSta_TurnLampFLThreCurr]  "<VHAL_DIDStaTurnLampFLThreCurr_raw>"
  bus_selector1/12 -> [u8_TurnLampFLThreCurr]  "<VHAL_TurnLampFLThreCurr_raw>"
  bus_selector1/13 -> [u8_DIDSta_TurnLampRLThreCurr]  "<VHAL_DIDStaTurnLampRLThreCurr_raw>"
  bus_selector1/14 -> [u8_TurnLampRLThreCurr]  "<VHAL_TurnLampRLThreCurr_raw>"
  bus_selector1/15 -> [u8_DIDSta_FMHTimer]  "<VHAL_DIDStaFMHTimer_raw>"
  bus_selector1/16 -> [u8_FMHTimer]  "<VHAL_FMHTimer_raw>"
  bus_selector1/17 -> [u8_DIDSta_AutoLock]  "<VHAL_DIDStaAutoLock_raw>"
  bus_selector1/18 -> [u8_AutoLock]  "<VHAL_AutoLock_raw>"
  bus_selector1/19 -> [u8_DIDSta_DRLDis]  "<VHAL_DIDStaDRLDis_raw>"
  bus_selector1/20 -> [u8_DRLDis]  "<VHAL_DRLDis_raw>"
  bus_selector1/21 -> [u8_DIDSta_AutoWipHSpdEN]  "<VHAL_DIDStaAutoWipHSpdEN_raw>"
  bus_selector1/22 -> [u8_AutoWipHSpdEN]  "<VHAL_AutoWipHSpdEN_raw>"
  bus_selector1/23 -> [u8_DIDSta_WipRLSCmdHoldFilter]  "<VHAL_DIDStaWipRLSCmdHoldFilter_raw>"
  bus_selector1/24 -> [u8_WipRLSCmdHoldFilter]  "<VHAL_WipRLSCmdHoldFilter_raw>"
  bus_selector1/25 -> [u8_DIDSta_WipRLSCmdCutFilter]  "<VHAL_DIDStaWipRLSCmdCutFilter_raw>"
  bus_selector1/26 -> [u8_WipRLSCmdCutFilter]  "<VHAL_WipRLSCmdCutFilter_raw>"
  bus_selector1/27 -> [u8_DIDSta_USSConfig]  "<VHAL_DIDStaUSSConfig_raw>"
  bus_selector1/28 -> [u8Array16_USSConfig]  "<VHAL_USSConfig_raw>"
  bus_selector1/29 -> [u8_DIDSta_TireSize]  "<VHAL_DIDStaTireSize_raw>"
  bus_selector1/30 -> [u8Array16_TireSize]  "<VHAL_TireSize_raw>"
  bus_selector1/31 -> [u8_DIDSta_APSFunConfig]  "<VHAL_DIDStaAPSFunConfig_raw>"
  bus_selector1/32 -> [u8Array16_APSFunConfig]  "<VHAL_APSFunConfig_raw>"
  bus_selector1/33 -> [u8_DIDSta_OBDReq]  "<VHAL_DIDStaOBDReq_raw>"
  bus_selector1/34 -> [u8_OBDReq]  "<VHAL_OBDReq_raw>"
  bus_selector1/35 -> [u8_DIDSta_TestGroup]  "<VHAL_DIDStaTestGroup_raw>"
  bus_selector1/36 -> [u8Array12_TestGroup]  "<VHAL_TestGroup_raw>"
  BHAL_DID_outputs/1 -> bus_selector1/1
  DIDLen/1 -> R_DIDWriteCDD_CSOP_DIDSet_XWDMode/1
  DIDNum/1 -> R_DIDWriteCDD_CSOP_DIDSet_XWDMode/2
  [u8_XWDMode] -> R_DIDWriteCDD_CSOP_DIDSet_XWDMode/3
  DIDLen1/1 -> R_DIDWriteCDD_CSOP_DIDSet_DKCKey/1
  DIDNum1/1 -> R_DIDWriteCDD_CSOP_DIDSet_DKCKey/2
  [u8Array8_DKCKey] -> R_DIDWriteCDD_CSOP_DIDSet_DKCKey/3
  DIDLen2/1 -> R_DIDWriteCDD_CSOP_DIDSet_DynoMode/1
  DIDNum2/1 -> R_DIDWriteCDD_CSOP_DIDSet_DynoMode/2
  [u8_DynoMode] -> R_DIDWriteCDD_CSOP_DIDSet_DynoMode/3
  DIDLen3/1 -> R_DIDWriteCDD_CSOP_DIDSet_APPPedalZP/1
  DIDNum3/1 -> R_DIDWriteCDD_CSOP_DIDSet_APPPedalZP/2
  [u8Array3_APPPedalZP] -> R_DIDWriteCDD_CSOP_DIDSet_APPPedalZP/3
  DIDLen4/1 -> R_DIDWriteCDD_CSOP_DIDSet_TurnLampFRThreCurr/1
  DIDNum4/1 -> R_DIDWriteCDD_CSOP_DIDSet_TurnLampFRThreCurr/2
  [u8_TurnLampFRThreCurr] -> R_DIDWriteCDD_CSOP_DIDSet_TurnLampFRThreCurr/3
  DIDLen5/1 -> R_DIDWriteCDD_CSOP_DIDSet_TurnLampRRThreCurr/1
  DIDNum5/1 -> R_DIDWriteCDD_CSOP_DIDSet_TurnLampRRThreCurr/2
  [u8_TurnLampRRThreCurr] -> R_DIDWriteCDD_CSOP_DIDSet_TurnLampRRThreCurr/3
  DIDLen6/1 -> R_DIDWriteCDD_CSOP_DIDSet_TurnLampFLThreCurr/1
  DIDNum6/1 -> R_DIDWriteCDD_CSOP_DIDSet_TurnLampFLThreCurr/2
  [u8_TurnLampFLThreCurr] -> R_DIDWriteCDD_CSOP_DIDSet_TurnLampFLThreCurr/3
  DIDLen7/1 -> R_DIDWriteCDD_CSOP_DIDSet_TurnLampRLThreCurr/1
  DIDNum7/1 -> R_DIDWriteCDD_CSOP_DIDSet_TurnLampRLThreCurr/2
  [u8_TurnLampRLThreCurr] -> R_DIDWriteCDD_CSOP_DIDSet_TurnLampRLThreCurr/3
  DIDLen8/1 -> R_DIDWriteCDD_CSOP_DIDSet_FMHTimer/1
  DIDNum8/1 -> R_DIDWriteCDD_CSOP_DIDSet_FMHTimer/2
  [u8_FMHTimer] -> R_DIDWriteCDD_CSOP_DIDSet_FMHTimer/3
  DIDLen9/1 -> R_DIDWriteCDD_CSOP_DIDSet_AutoLock/1
  DIDNum9/1 -> R_DIDWriteCDD_CSOP_DIDSet_AutoLock/2
  [u8_AutoLock] -> R_DIDWriteCDD_CSOP_DIDSet_AutoLock/3
  DIDLen10/1 -> R_DIDWriteCDD_CSOP_DIDSet_DRLDis/1
  DIDNum10/1 -> R_DIDWriteCDD_CSOP_DIDSet_DRLDis/2
  [u8_DRLDis] -> R_DIDWriteCDD_CSOP_DIDSet_DRLDis/3
  DIDLen11/1 -> R_DIDWriteCDD_CSOP_DIDSet_AutoWipHSpdEN/1
  DIDNum11/1 -> R_DIDWriteCDD_CSOP_DIDSet_AutoWipHSpdEN/2
  [u8_AutoWipHSpdEN] -> R_DIDWriteCDD_CSOP_DIDSet_AutoWipHSpdEN/3
  DIDLen12/1 -> R_DIDWriteCDD_CSOP_DIDSet_WipRLSCmdHoldFilter/1
  DIDNum12/1 -> R_DIDWriteCDD_CSOP_DIDSet_WipRLSCmdHoldFilter/2
  [u8_WipRLSCmdHoldFilter] -> R_DIDWriteCDD_CSOP_DIDSet_WipRLSCmdHoldFilter/3
  DIDLen13/1 -> R_DIDWriteCDD_CSOP_DIDSet_WipRLSCmdCutFilter/1
  DIDNum13/1 -> R_DIDWriteCDD_CSOP_DIDSet_WipRLSCmdCutFilter/2
  [u8_WipRLSCmdCutFilter] -> R_DIDWriteCDD_CSOP_DIDSet_WipRLSCmdCutFilter/3
  DIDLen14/1 -> R_DIDWriteCDD_CSOP_DIDSet_LFSensorID/1
  DIDNum14/1 -> R_DIDWriteCDD_CSOP_DIDSet_LFSensorID/2
  [u8Array4_LFSensorID] -> R_DIDWriteCDD_CSOP_DIDSet_LFSensorID/3
  DIDLen15/1 -> R_DIDWriteCDD_CSOP_DIDSet_RFSensorID/1
  DIDNum15/1 -> R_DIDWriteCDD_CSOP_DIDSet_RFSensorID/2
  [u8Array4_RFSensorID] -> R_DIDWriteCDD_CSOP_DIDSet_RFSensorID/3
  DIDLen16/1 -> R_DIDWriteCDD_CSOP_DIDSet_LRSensorID/1
  DIDNum16/1 -> R_DIDWriteCDD_CSOP_DIDSet_LRSensorID/2
  [u8Array4_LRSensorID] -> R_DIDWriteCDD_CSOP_DIDSet_LRSensorID/3
  DIDLen17/1 -> R_DIDWriteCDD_CSOP_DIDSet_RRSensorID/1
  DIDNum17/1 -> R_DIDWriteCDD_CSOP_DIDSet_RRSensorID/2
  [u8Array4_RRSensorID] -> R_DIDWriteCDD_CSOP_DIDSet_RRSensorID/3
  DIDLen18/1 -> R_DIDWriteCDD_CSOP_DIDSet_WhlPres/1
  DIDNum18/1 -> R_DIDWriteCDD_CSOP_DIDSet_WhlPres/2
  [u8Array4_WhlPres] -> R_DIDWriteCDD_CSOP_DIDSet_WhlPres/3
  DIDLen19/1 -> R_DIDWriteCDD_CSOP_DIDSet_WhlTmp/1
  DIDNum19/1 -> R_DIDWriteCDD_CSOP_DIDSet_WhlTmp/2
  [u8Array4_WhlTmp] -> R_DIDWriteCDD_CSOP_DIDSet_WhlTmp/3
  DIDLen20/1 -> R_DIDWriteCDD_CSOP_DIDSet_WhlSensorBattSta/1
  DIDNum20/1 -> R_DIDWriteCDD_CSOP_DIDSet_WhlSensorBattSta/2
  [u8_WhlSensorBattSta] -> R_DIDWriteCDD_CSOP_DIDSet_WhlSensorBattSta/3
  DIDLen21/1 -> R_DIDWriteCDD_CSOP_DIDSet_LFLowPresThre/1
  DIDNum21/1 -> R_DIDWriteCDD_CSOP_DIDSet_LFLowPresThre/2
  [u8_LFLowPresThre] -> R_DIDWriteCDD_CSOP_DIDSet_LFLowPresThre/3
  DIDLen22/1 -> R_DIDWriteCDD_CSOP_DIDSet_RFLowPresThre/1
  DIDNum22/1 -> R_DIDWriteCDD_CSOP_DIDSet_RFLowPresThre/2
  [u8_RFLowPresThre] -> R_DIDWriteCDD_CSOP_DIDSet_RFLowPresThre/3
  DIDLen23/1 -> R_DIDWriteCDD_CSOP_DIDSet_LRLowPresThre/1
  DIDNum23/1 -> R_DIDWriteCDD_CSOP_DIDSet_LRLowPresThre/2
  [u8_LRLowPresThre] -> R_DIDWriteCDD_CSOP_DIDSet_LRLowPresThre/3
  DIDLen24/1 -> R_DIDWriteCDD_CSOP_DIDSet_RRLowPresThre/1
  DIDNum24/1 -> R_DIDWriteCDD_CSOP_DIDSet_RRLowPresThre/2
  [u8_RRLowPresThre] -> R_DIDWriteCDD_CSOP_DIDSet_RRLowPresThre/3
  DIDLen25/1 -> R_DIDWriteCDD_CSOP_DIDSet_SensorMode/1
  DIDNum25/1 -> R_DIDWriteCDD_CSOP_DIDSet_SensorMode/2
  [u8_SensorMode] -> R_DIDWriteCDD_CSOP_DIDSet_SensorMode/3
  DIDLen26/1 -> R_DIDWriteCDD_CSOP_DIDSet_TPMSLearnSta/1
  DIDNum26/1 -> R_DIDWriteCDD_CSOP_DIDSet_TPMSLearnSta/2
  [u8_TPMSLearnSta] -> R_DIDWriteCDD_CSOP_DIDSet_TPMSLearnSta/3
  DIDLen27/1 -> R_DIDWriteCDD_CSOP_DIDSet_USSConfig/1
  DIDNum27/1 -> R_DIDWriteCDD_CSOP_DIDSet_USSConfig/2
  [u8Array16_USSConfig] -> R_DIDWriteCDD_CSOP_DIDSet_USSConfig/3
  DIDLen28/1 -> R_DIDWriteCDD_CSOP_DIDSet_TireSize/1
  DIDNum28/1 -> R_DIDWriteCDD_CSOP_DIDSet_TireSize/2
  [u8Array16_TireSize] -> R_DIDWriteCDD_CSOP_DIDSet_TireSize/3
  DIDLen29/1 -> R_DIDWriteCDD_CSOP_DIDSet_APSFunConfig/1
  DIDNum29/1 -> R_DIDWriteCDD_CSOP_DIDSet_APSFunConfig/2
  [u8Array16_APSFunConfig] -> R_DIDWriteCDD_CSOP_DIDSet_APSFunConfig/3
  DIDLen30/1 -> R_DIDWriteCDD_CSOP_DIDSet_VSS/1
  DIDNum30/1 -> R_DIDWriteCDD_CSOP_DIDSet_VSS/2
  [u8_VSS] -> R_DIDWriteCDD_CSOP_DIDSet_VSS/3
  DIDLen31/1 -> R_DIDWriteCDD_CSOP_DIDSet_OBDReq/1
  DIDNum31/1 -> R_DIDWriteCDD_CSOP_DIDSet_OBDReq/2
  [u8_OBDReq] -> R_DIDWriteCDD_CSOP_DIDSet_OBDReq/3
  DIDLen32/1 -> R_DIDWriteCDD_CSOP_DIDSet_RUNTM/1
  DIDNum32/1 -> R_DIDWriteCDD_CSOP_DIDSet_RUNTM/2
  [u8Array2_RUNTM] -> R_DIDWriteCDD_CSOP_DIDSet_RUNTM/3
  DIDLen33/1 -> R_DIDWriteCDD_CSOP_DIDSet_MILDIST/1
  DIDNum33/1 -> R_DIDWriteCDD_CSOP_DIDSet_MILDIST/2
  [u8Array2_MILDIST] -> R_DIDWriteCDD_CSOP_DIDSet_MILDIST/3
  DIDLen34/1 -> R_DIDWriteCDD_CSOP_DIDSet_CLRDIST/1
  DIDNum34/1 -> R_DIDWriteCDD_CSOP_DIDSet_CLRDIST/2
  [u8Array2_CLRDIST] -> R_DIDWriteCDD_CSOP_DIDSet_CLRDIST/3
  DIDLen35/1 -> R_DIDWriteCDD_CSOP_DIDSet_APPD/1
  DIDNum35/1 -> R_DIDWriteCDD_CSOP_DIDSet_APPD/2
  [u8_APPD] -> R_DIDWriteCDD_CSOP_DIDSet_APPD/3
  DIDLen36/1 -> R_DIDWriteCDD_CSOP_DIDSet_APPE/1
  DIDNum36/1 -> R_DIDWriteCDD_CSOP_DIDSet_APPE/2
  [u8_APPE] -> R_DIDWriteCDD_CSOP_DIDSet_APPE/3
  DIDLen37/1 -> R_DIDWriteCDD_CSOP_DIDSet_ODOMETER/1
  DIDNum37/1 -> R_DIDWriteCDD_CSOP_DIDSet_ODOMETER/2
  [u8Array4_ODOMETER] -> R_DIDWriteCDD_CSOP_DIDSet_ODOMETER/3
  DIDLen38/1 -> R_DIDWriteCDD_CSOP_DIDSet_NUMPSATRIPSFLTMEMCLR/1
  DIDNum38/1 -> R_DIDWriteCDD_CSOP_DIDSet_NUMPSATRIPSFLTMEMCLR/2
  [u8Array2_NUMPSATRIPSFLTMEMCLR] -> R_DIDWriteCDD_CSOP_DIDSet_NUMPSATRIPSFLTMEMCLR/3
  DIDLen39/1 -> R_DIDWriteCDD_CSOP_DIDSet_VIN/1
  DIDNum39/1 -> R_DIDWriteCDD_CSOP_DIDSet_VIN/2
  [u8Array17_VIN] -> R_DIDWriteCDD_CSOP_DIDSet_VIN/3
  DIDLen40/1 -> R_DIDWriteCDD_CSOP_DIDSet_CALID/1
  DIDNum40/1 -> R_DIDWriteCDD_CSOP_DIDSet_CALID/2
  [u8Array16_CALID] -> R_DIDWriteCDD_CSOP_DIDSet_CALID/3
  DIDLen41/1 -> R_DIDWriteCDD_CSOP_DIDSet_ECUNAME/1
  DIDNum41/1 -> R_DIDWriteCDD_CSOP_DIDSet_ECUNAME/2
  [u8Array20_ECUNAME] -> R_DIDWriteCDD_CSOP_DIDSet_ECUNAME/3
  DIDLen42/1 -> R_DIDWriteCDD_CSOP_DIDSet_ProtocolId/1
  DIDNum42/1 -> R_DIDWriteCDD_CSOP_DIDSet_ProtocolId/2
  [u8_ProtocolId] -> R_DIDWriteCDD_CSOP_DIDSet_ProtocolId/3
  DIDLen43/1 -> R_DIDWriteCDD_CSOP_DIDSet_TestGroup/1
  DIDNum43/1 -> R_DIDWriteCDD_CSOP_DIDSet_TestGroup/2
  [u8Array12_TestGroup] -> R_DIDWriteCDD_CSOP_DIDSet_TestGroup/3
  DIDLen44/1 -> R_DIDWriteCDD_CSOP_DIDSet_PSA/1
  DIDNum44/1 -> R_DIDWriteCDD_CSOP_DIDSet_PSA/2
  [u8Array24_PSA] -> R_DIDWriteCDD_CSOP_DIDSet_PSA/3
  DIDLen45/1 -> R_DIDWriteCDD_CSOP_DIDSet_PKE/1
  DIDNum45/1 -> R_DIDWriteCDD_CSOP_DIDSet_PKE/2
  [u8Array8_PKE] -> R_DIDWriteCDD_CSOP_DIDSet_PKE/3
  DIDLen46/1 -> R_DIDWriteCDD_CSOP_DIDSet_CDEODT/1
  DIDNum46/1 -> R_DIDWriteCDD_CSOP_DIDSet_CDEODT/2
  [u8Array8_CDEODT] -> R_DIDWriteCDD_CSOP_DIDSet_CDEODT/3
  DIDLen47/1 -> R_DIDWriteCDD_CSOP_DIDSet_QTYPSATRIPS/1
  DIDNum47/1 -> R_DIDWriteCDD_CSOP_DIDSet_QTYPSATRIPS/2
  [u8Array8_QTYPSATRIPS] -> R_DIDWriteCDD_CSOP_DIDSet_QTYPSATRIPS/3
  DIDLen48/1 -> R_DIDWriteCDD_CSOP_DIDSet_DKCSta/1
  DIDNum48/1 -> R_DIDWriteCDD_CSOP_DIDSet_DKCSta/2
  [u8Array2_DKCSta] -> R_DIDWriteCDD_CSOP_DIDSet_DKCSta/3
  DIDLen49/1 -> R_DIDWriteCDD_CSOP_DIDSet_DKCBLESta/1
  DIDNum49/1 -> R_DIDWriteCDD_CSOP_DIDSet_DKCBLESta/2
  [u8Array2_DKCBLESta] -> R_DIDWriteCDD_CSOP_DIDSet_DKCBLESta/3
  DIDLen50/1 -> R_DIDWriteCDD_CSOP_DIDSet_UWBAnchorSta/1
  DIDNum50/1 -> R_DIDWriteCDD_CSOP_DIDSet_UWBAnchorSta/2
  [u8Array93_UWBAnchorSta] -> R_DIDWriteCDD_CSOP_DIDSet_UWBAnchorSta/3
  DIDLen51/1 -> R_DIDWriteCDD_CSOP_DIDSet_LIDAAnchorSta/1
  DIDNum51/1 -> R_DIDWriteCDD_CSOP_DIDSet_LIDAAnchorSta/2
  [u8Array21_LIDAAnchorSta] -> R_DIDWriteCDD_CSOP_DIDSet_LIDAAnchorSta/3
  DIDLen52/1 -> R_DIDWriteCDD_CSOP_DIDSet_DoorNFCAnchorSta/1
  DIDNum52/1 -> R_DIDWriteCDD_CSOP_DIDSet_DoorNFCAnchorSta/2
  [u8Array21_DoorNFCAnchorSta] -> R_DIDWriteCDD_CSOP_DIDSet_DoorNFCAnchorSta/3
  DIDLen53/1 -> R_DIDWriteCDD_CSOP_DIDSet_UIDSta/1
  DIDNum53/1 -> R_DIDWriteCDD_CSOP_DIDSet_UIDSta/2
  [u8Array26_UIDSta] -> R_DIDWriteCDD_CSOP_DIDSet_UIDSta/3
  DIDLen54/1 -> R_DIDWriteCDD_CSOP_DIDSet_FDDKCCoordXY/1
  DIDNum54/1 -> R_DIDWriteCDD_CSOP_DIDSet_FDDKCCoordXY/2
  [u8Array3_FDDKCCoordXY] -> R_DIDWriteCDD_CSOP_DIDSet_FDDKCCoordXY/3

== system SWC_HALOUT_type/run_SWC_HALOUT_Tx_5ms_sys/HALOUT_AFTER ==
  E2E_CAN3_VCU1_Trigger : Inport
  E2E_CAN3_VCU1_Trigger_toNIDEC : Inport  Port=2
  E2E_CAN4_VCU1_Trigger : Inport  Port=3
  function : TriggerPort  TriggerType=function-call  VariantControl=(inherit)  PortDimensions=1
  R_E2E_CAN3_VCU1_CSOP_Write_CAN3_VCU1 : Subsystem
  R_E2E_CAN3_VCU1_toNIDEC_CSOP_Write_CAN3_VCU1_toNIDEC : Subsystem
  R_E2E_CAN4_VCU1_CSOP_Write_CAN4_VCU1 : Subsystem
  wires:
  E2E_CAN3_VCU1_Trigger/1 -> R_E2E_CAN3_VCU1_CSOP_Write_CAN3_VCU1/Enable
  E2E_CAN3_VCU1_Trigger_toNIDEC/1 -> R_E2E_CAN3_VCU1_toNIDEC_CSOP_Write_CAN3_VCU1_toNIDEC/Enable
  E2E_CAN4_VCU1_Trigger/1 -> R_E2E_CAN4_VCU1_CSOP_Write_CAN4_VCU1/Enable

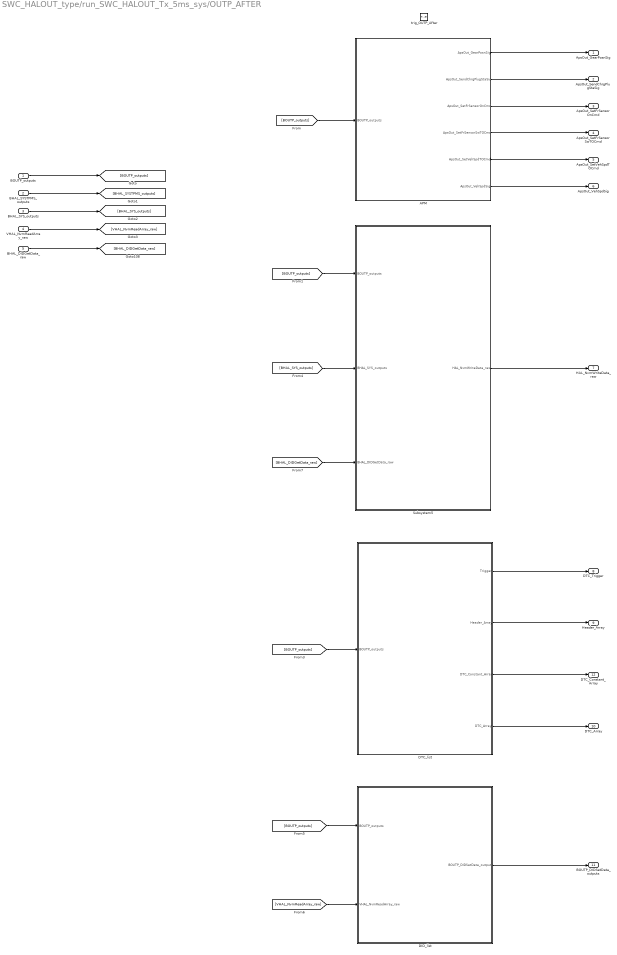
== system SWC_HALOUT_type/run_SWC_HALOUT_Tx_5ms_sys/OUTP_AFTER ==
  BOUTP_outputs : Inport
  BHAL_SYSTPMS_outputs : Inport  Port=2
  BHAL_SYS_outputs : Inport  Port=3
  VHAL_NvmReadArray_raw : Inport  Port=4
  BHAL_DIDGetData_raw : Inport  Port=5
  trig_OUTP_After : TriggerPort  TriggerType=function-call  VariantControl=(inherit)
  APM : Subsystem
  DID_list : Subsystem
  DTC_list : Subsystem
  Subsystem5 : Subsystem
  ApsOut_GearPosnSig : Outport
  ApsOut_SendChrgPlugStaSig : Outport  Port=2
  ApsOut_SetFrSensorOnCmd : Outport  Port=3
  ApsOut_SetFrSensorSwTOCmd : Outport  Port=4
  ApsOut_SetVehSpdTOCmd : Outport  Port=5
  ApsOut_VehSpdSig : Outport  Port=6
  HAL_NvmWriteData_raw : Outport  Port=7
  DTC_Trigger : Outport  Port=8
  Header_Array : Outport  Port=9
  DTC_Array : Outport  Port=10
  BOUTP_DIDSetData_outputs : Outport  Port=11
  DTC_Constant_Array : Outport  Port=12
  wires:
  APM/1(ApsOut_GearPosnSig) -> ApsOut_GearPosnSig/1
  Subsystem5/1(HAL_NvmWriteData_raw) -> HAL_NvmWriteData_raw/1
  APM/2(ApsOut_SendChrgPlugStaSig) -> ApsOut_SendChrgPlugStaSig/1
  APM/5(ApsOut_SetVehSpdTOCmd) -> ApsOut_SetVehSpdTOCmd/1
  APM/3(ApsOut_SetFrSensorOnCmd) -> ApsOut_SetFrSensorOnCmd/1
  BOUTP_outputs/1 -> [BOUTP_outputs]
  APM/6(ApsOut_VehSpdSig) -> ApsOut_VehSpdSig/1
  APM/4(ApsOut_SetFrSensorSwTOCmd) -> ApsOut_SetFrSensorSwTOCmd/1
  [BOUTP_outputs] -> APM/1(BOUTP_outputs)
  [BOUTP_outputs] -> Subsystem5/1(BOUTP_outputs)
  BHAL_SYSTPMS_outputs/1 -> [BHAL_SYSTPMS_outputs]
  [BOUTP_outputs] -> DTC_list/1(BOUTP_outputs)
  DTC_list/1(Trigger) -> DTC_Trigger/1
  DTC_list/2(Header_Array) -> Header_Array/1
  BHAL_SYS_outputs/1 -> [BHAL_SYS_outputs]
  [BHAL_SYS_outputs] -> Subsystem5/2(BHAL_SYS_outputs)
  [BOUTP_outputs] -> DID_list/1(BOUTP_outputs)
  DID_list/1(BOUTP_DIDSetData_outputs) -> BOUTP_DIDSetData_outputs/1
  [VHAL_NvmReadArray_raw] -> DID_list/2(VHAL_NvmReadArray_raw)
  BHAL_DIDGetData_raw/1 -> [BHAL_DIDGetData_raw]
  VHAL_NvmReadArray_raw/1 -> [VHAL_NvmReadArray_raw]
  [BHAL_DIDGetData_raw] -> Subsystem5/3(BHAL_DIDGetData_raw)
  DTC_list/4(DTC_Array) -> DTC_Array/1
  DTC_list/3(DTC_Constant_Array) -> DTC_Constant_Array/1

== system SWC_HALOUT_type/run_SWC_HALOUT_Tx_5ms_sys/R_DIDWriteCDD_CSOP_DIDSet_NVMPedalZP ==
  In3 : Inport
  Enable : EnablePort
  DIDLen7 : Constant  Value=DIDNum_NVMPedalZP
  DIDNum7 : Constant  Value=DIDLen_NVMPedalZP
  R_DIDWriteCDD_CSOP_DIDSet_NVMPedalZP : FunctionCaller  FunctionPrototype=R_DIDWriteCDD_CSOP_DIDSet_NVMPedalZP(u16_DIDNum_NVMPedalZP,u16_DIDLen_NVMPedalZP,u8Array3_NVMPedalZP)  InputArgumentSpecifications=uint16(1), uint16(1), uint8([1;1;1])
  wires:
  In3/1 -> R_DIDWriteCDD_CSOP_DIDSet_NVMPedalZP/3
  DIDNum7/1 -> R_DIDWriteCDD_CSOP_DIDSet_NVMPedalZP/2
  DIDLen7/1 -> R_DIDWriteCDD_CSOP_DIDSet_NVMPedalZP/1

== system SWC_HALOUT_type/run_SWC_HALOUT_Tx_5ms_sys/R_FDCCDD_Inner_CSOP_FDC_AppCallSleep ==
  Enable : EnablePort
  R_FDCCDD_Inner_CSOP_FDC_AppCallSleep : FunctionCaller  FunctionPrototype=R_FDCCDD_Inner_CSOP_FDC_AppCallSleep()

== system SWC_HALOUT_type/run_SWC_HALOUT_Tx_5ms_sys/R_HALOUTCDD_CSOP_AppNmStateReq ==
  WakeReq : Inport
  SleepReq : Inport  Port=2
  Enable : EnablePort
  R_HALOUTCDD_CSOP_AppNmStateReq : FunctionCaller  FunctionPrototype=R_HALOUTCDD_CSOP_AppNmStateReq(u8_WakeUpReq,u8_SleepReq)  InputArgumentSpecifications=uint8(1), uint8(1)
  wires:
  WakeReq/1 -> R_HALOUTCDD_CSOP_AppNmStateReq/1
  SleepReq/1 -> R_HALOUTCDD_CSOP_AppNmStateReq/2

== system SWC_HALOUT_type/run_SWC_HALOUT_Tx_5ms_sys/R_HALOUTCDD_CSOP_ResetPedalZeroPosDone ==
  Enable : EnablePort
  R_HALOUTCDD_CSOP_ResetPedalZeroPosDone : FunctionCaller  FunctionPrototype=R_HALOUTCDD_CSOP_ResetPedalZeroPosDone()

== system SWC_HALOUT_type/run_SWC_HALOUT_Tx_5ms_sys/R_HALOUTCDD_CSOP_SetAcoreRebootCmdACK ==
  Enable : EnablePort
  R_HALOUTCDD_CSOP_SetAcoreRebootCmdACK : FunctionCaller  FunctionPrototype=R_HALOUTCDD_CSOP_SetAcoreRebootCmdACK()

== system SWC_HALOUT_type/run_SWC_HALOUT_Tx_5ms_sys/R_HALOUTCDD_CSOP_SleepRequest ==
  SleepState : Inport
  WakeUpTime : Inport  Port=2
  Enable : EnablePort
  R_HALOUTCDD_CSOP_SleepRequest : FunctionCaller  FunctionPrototype=R_HALOUTCDD_CSOP_SleepRequest(u32_SleepyState,u32_Wakeup_Timer_s)  InputArgumentSpecifications=uint32(1), uint32(1)
  wires:
  WakeUpTime/1 -> R_HALOUTCDD_CSOP_SleepRequest/2
  SleepState/1 -> R_HALOUTCDD_CSOP_SleepRequest/1

== system SWC_HALOUT_type/run_SWC_HALOUT_Tx_5ms_sys/R_HALOUTCDD_CSOP_TPMSSensorIDRegSetResults ==
  In1 : Inport
  Enable : EnablePort
  R_HALOUTCDD_CSOP_TPMSSensorIDRegSetResults : FunctionCaller  FunctionPrototype=R_HALOUTCDD_CSOP_TPMSSensorIDRegSetResults(u8Array2_TPMSSensorIDRegResults)  InputArgumentSpecifications=uint8([1;1])
  wires:
  In1/1 -> R_HALOUTCDD_CSOP_TPMSSensorIDRegSetResults/1

== system SWC_HALOUT_type/run_SWC_HALOUT_Tx_5ms_sys/R_IOExpOUT_CDD_CSOP_IOExpSetVal ==
  In1 : Inport
  Enable : EnablePort
  R_IOExpOUT_CDD_CSOP_IOExpSetVal : FunctionCaller  FunctionPrototype=R_IOExpOUT_CDD_CSOP_IOExpSetVal(u8_IVIRstCmd)  InputArgumentSpecifications=uint8(1)
  wires:
  In1/1 -> R_IOExpOUT_CDD_CSOP_IOExpSetVal/1

== system SWC_HALOUT_type/run_SWC_HALOUT_Tx_5ms_sys/R_NVMWriteCDD_Inner_NVM_WriteOperation ==
  Enable : EnablePort
  R_NVMWriteCDD_Inner_NVM_WriteOperation : FunctionCaller  FunctionPrototype=R_NVMWriteCDD_Inner_NVM_WriteOperation()

== system SWC_HALOUT_type/run_SWC_HALOUT_Tx_5ms_sys/R_UDSCDD_CSOP_DdmRestartOperationCycle ==
  Enable : EnablePort
  R_UDSCDD_CSOP_DdmRestartOperationCycle : FunctionCaller  FunctionPrototype=R_UDSCDD_CSOP_DdmRestartOperationCycle()

== system SWC_HALOUT_type/run_SWC_HALOUT_Tx_5ms_sys/R_UDSCDD_CSOP_SetDTCStatus ==
  Header_Array : Inport
  DTC_Array : Inport  Port=2
  In3 : Inport  Port=3
  Enable : EnablePort
  R_UDSCDD_CSOP_SetDTCStatus : FunctionCaller  FunctionPrototype=u8_ReturnStatus = R_UDSCDD_CSOP_SetDTCStatus(u32Array10_Header,u32Array320_DTC,u16Array320_DTCConst)  InputArgumentSpecifications=uint32([1;1;1;1;1;1;1;1;1;1]), uint32([1;1;1;1;1;1;1;1;1;1;1;1;1;1;1;1;1;1;1;1;1;1;1;1;1;1;1;1;1;1;1;1;1;1;1;1;1;1;1;1;1;1;1;1;1;1;1;1;1;1;1;1;1;1;1;1;1;1;1;1;1;1;1;1;1;1;1;1;1;1;1;1;1;1;1;1;1;1;1;1;1;1;1;1;1;1;1;1;1;1;1;1;1;1;1;1;1;1;1;1;1;1;1;1;1;1;1;1;1;1;1;1;1;1;1;1;1;1;1;1;1;1;1;1;1;1;1;1;1;1;1;1;1;1;1;1;1;1;1;1;1;1;1;1;1;1;1;1;1;1;1;1;1;1;1;1;1;1;1;1;1;1;1;1;1;1;1;1;1;1;1;1;1;1;1;1;1;1;1;1;1;1;1;1;1;1;1;1;1;1;1;1;1;1;1;1;1;1;1;1;1;1;1;1;1;1;1;1;1;1;1;1;1;1;1;1;1;1;1;1;1;1;1;1;1;1;1;1;1;1;1;1;1;1;1;1;1;1;1;1;1;1;1;1;1;1;1;1;1;1;1;1;1;1;1;1;1;1;1;1;1;1;1;1;1;1;1;1;1;1;1;1;1;1;1;1;1;1;1;1;1;1;1;1;1;1;1;1;1;1;1;1;1;1;1;1;1;1;1;1;1;1;1;1;1;1;1;1;1;1;1;1;1;1;1;1;1;1;1;1]), uint16([1;1;1;1;1;1;1;1;1;1;1;1;1;1;1;1;1;1;1;1;1;1;1;1;1;1;1;1;1;1;1;1;1;1;1;1;1;1;1;1;1;1;1;1;1;1;1;1;1;1;1;1;1;1;1;1;1;1;1;1;1;1;1;1;1;1;1;1;1;1;1;1;1;1;1;1;1;1;1;1;1;1;1;1;1;1;1;1;1;1;1;1;1;1;1;1;1;1;1;1;1;1;1;1;1;1;1;1;1;1;1;1;1;1;1;1;1;1;1;1;1;1;1;1;1;1;1;1;1;1;1;1;1;1;1;1;1;1;1;1;1;1;1;1;1;1;1;1;1;1;1;1;1;1;1;1;1;1;1;1;1;1;1;1;1;1;1;1;1;1;1;1;1;1;1;1;1;1;1;1;1;1;1;1;1;1;1;1;1;1;1;1;1;1;1;1;1;1;1;1;1;1;1;1;1;1;1;1;1;1;1;1;1;1;1;1;1;1;1;1;1;1;1;1;1;1;1;1;1;1;1;1;1;1;1;1;1;1;1;1;1;1;1;1;1;1;1;1;1;1;1;1;1;1;1;1;1;1;1;1;1;1;1;1;1;1;1;1;1;1;1;1;1;1;1;1;1;1;1;1;1;1;1;1;1;1;1;1;1;1;1;1;1;1;1;1;1;1;1;1;1;1;1;1;1;1;1;1;1;1;1;1;1;1;1;1;1;1;1;1])  OutputArgumentSpecifications=uint8(1)
  Out1 : Outport
  wires:
  DTC_Array/1 -> R_UDSCDD_CSOP_SetDTCStatus/2
  In3/1 -> R_UDSCDD_CSOP_SetDTCStatus/3
  Header_Array/1 -> R_UDSCDD_CSOP_SetDTCStatus/1
  R_UDSCDD_CSOP_SetDTCStatus/1 -> Out1/1

== system SWC_HALOUT_type/run_SWC_HALOUT_Tx_5ms_sys/R_WDGCDD_CSOP_Call_WDG_AppEnd ==
  Enable : EnablePort
  R_WDGCDD_CSOP_Call_WDG_AppEnd : FunctionCaller  FunctionPrototype=R_WDGCDD_CSOP_Call_WDG_AppEnd()

== system SWC_HALOUT_type/run_SWC_HALOUT_Tx_5ms_sys/HALOUT_AFTER/R_E2E_CAN3_VCU1_CSOP_Write_CAN3_VCU1 ==
  Enable : EnablePort
  R_E2E_CAN3_VCU1_CSOP_Write_CAN3_VCU1 : FunctionCaller  FunctionPrototype=R_E2E_CAN3_VCU1_CSOP_Write_CAN3_VCU1()

== system SWC_HALOUT_type/run_SWC_HALOUT_Tx_5ms_sys/HALOUT_AFTER/R_E2E_CAN3_VCU1_toNIDEC_CSOP_Write_CAN3_VCU1_toNIDEC ==
  In1 : EnablePort
  R_E2E_CAN3_VCU1_toNIDEC_CSOP_Write_CAN3_VCU1_toNIDEC : FunctionCaller  FunctionPrototype=R_E2E_CAN3_VCU1_toNIDEC_CSOP_Write_CAN3_VCU1_toNIDEC()

== system SWC_HALOUT_type/run_SWC_HALOUT_Tx_5ms_sys/HALOUT_AFTER/R_E2E_CAN4_VCU1_CSOP_Write_CAN4_VCU1 ==
  In1 : EnablePort
  R_E2E_CAN4_VCU1_CSOP_Write_CAN4_VCU1 : FunctionCaller  FunctionPrototype=R_E2E_CAN4_VCU1_CSOP_Write_CAN4_VCU1()

== system SWC_HALOUT_type/run_SWC_HALOUT_Tx_5ms_sys/OUTP_AFTER/APM ==
  BOUTP_outputs : Inport  OutDataTypeStr=Bus: BOUTP_outputs
  Bus Selector : BusSelector  OutputSignals=VOUTP_VehSpeed_kph,VOUTP_ShiftGearPosn_enum,VOUTP_FSOffSw_enum,VOUTP_VehSpeedTimeOut_flg,VOUTP_FSOffSwTimeOut_flg,VOUTP_ChrgPlugSta_enum
  Data Type Conversion : DataTypeConversion  OutDataTypeStr=single
  Data Type Conversion{1..5} (5 alike) : DataTypeConversion  OutDataTypeStr=uint8
  ApsOut_GearPosnSig : Outport
  ApsOut_SendChrgPlugStaSig : Outport  Port=2
  ApsOut_SetFrSensorOnCmd : Outport  Port=3
  ApsOut_SetFrSensorSwTOCmd : Outport  Port=4
  ApsOut_SetVehSpdTOCmd : Outport  Port=5
  ApsOut_VehSpdSig : Outport  Port=6
  wires:
  BOUTP_outputs/1 -> [BOUTP_outputs]
  [BOUTP_outputs] -> Bus Selector/1
  Bus Selector/1 -> Data Type Conversion/1  "<VOUTP_VehSpeed_kph>"
  Bus Selector/2 -> Data Type Conversion1/1  "<VOUTP_ShiftGearPosn_enum>"
  Bus Selector/3 -> Data Type Conversion2/1  "<VOUTP_FSOffSw_enum>"
  Bus Selector/4 -> Data Type Conversion3/1  "<VOUTP_VehSpeedTimeOut_flg>"
  Bus Selector/5 -> Data Type Conversion4/1  "<VOUTP_FSOffSwTimeOut_flg>"
  Data Type Conversion1/1 -> ApsOut_GearPosnSig/1
  Data Type Conversion2/1 -> ApsOut_SetFrSensorOnCmd/1
  Data Type Conversion4/1 -> ApsOut_SetFrSensorSwTOCmd/1
  Data Type Conversion5/1 -> ApsOut_SendChrgPlugStaSig/1
  Bus Selector/6 -> Data Type Conversion5/1  "<VOUTP_ChrgPlugSta_enum>"
  Data Type Conversion/1 -> ApsOut_VehSpdSig/1
  Data Type Conversion3/1 -> ApsOut_SetVehSpdTOCmd/1
